simulink model "Pacemaker_model_assgn2"  (R2019a)
settings: Solver=FixedStepAuto  StartTime=0.0  StopTime=inf  FixedStep=1e-3  RelTol=1e-3  EnableMultiTasking=on
undefined symbols (not defined in the file): D0, D1, D10, D11, D12, D13, D2, D3, D4, D5, D6, D7, D8, D9, PTA0, PTA1, PTA2, PTB23, PTB9, PTC16, PTC17, PTC2, PTC3, PTC4, PTD0, PTD1, PTD2, PTD3
libraries: frdmk64flib x21, etargetslib x15, dspstat3 x1
settings Model: ExtModeTrigDuration=5  Creator=dr_pa  LastModifiedBy=dr_pa
settings SolverCC: ConcurrentTasks=on
settings OptimizationCC: EnhancedBackFolding=on  PassReuseOutputArgsAs=Individual arguments  MaxStackSize=64  OptimizeBlockOrder=speed  DifferentSizesBufferReuse=on  OptimizationCustomize=off
settings DebuggingCC: ParameterTunabilityLossMsg=error
settings HardwareCC: ProdBitPerPointer=32  ProdBitPerSizeT=32  ProdBitPerPtrDiffT=32  ProdLargestAtomicInteger=Long  ProdLargestAtomicFloat=Double  ProdWordSize=32  ProdHWDeviceType=ARM Compatible->ARM Cortex
settings SFSimCC: MATLABDynamicMemAlloc=off
settings RTWCC: SystemTargetFile=ert.tlc  HardwareBoard=NXP FRDM-K64F  TLCOptions="-aInlineSetEventsForThisBaseRateFcn=TLC_FALSE -aSuppressMultiTaskScheduler=TLC_FALSE  -aRateBasedStepFcn=0"  TemplateMakefile=ert_default_tmf  GenerateReport=on  Toolchain=GNU Tools for ARM Embedded Processors  BuildConfiguration=Faster Runs  IncludeHyperlinkInReport=on  LaunchReport=on  GenerateTraceInfo=on  GenerateTraceReport=on  GenerateTraceReportSl=on  GenerateTraceReportSf=on  GenerateTraceReportEml=on
settings CodeAppCC: ForceParamTrailComments=on  IgnoreCustomStorageClasses=off  OperatorAnnotations=on  SimulinkDataObjDesc=on  SFDataObjDesc=on  InsertBlockDesc=on

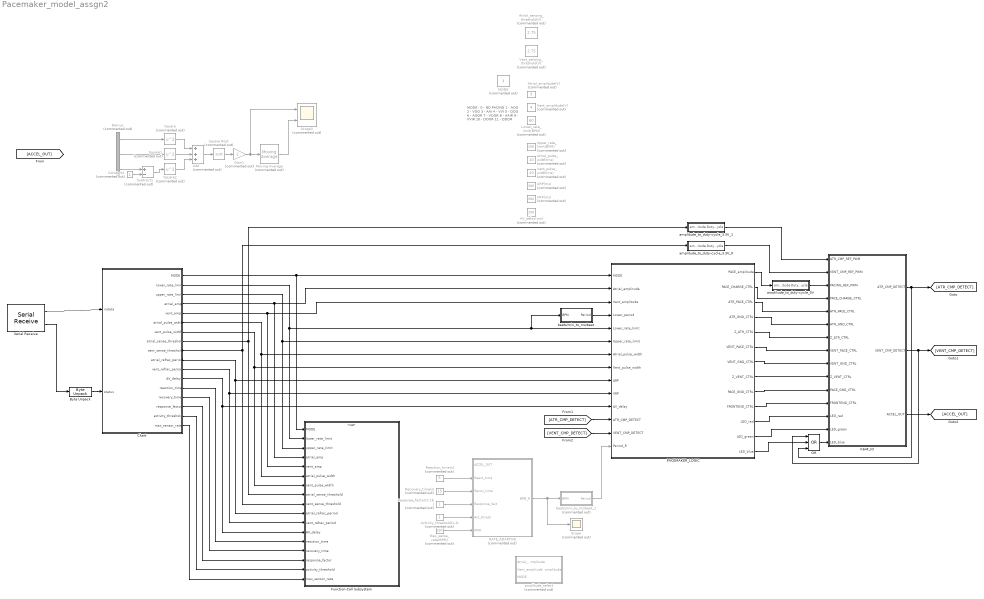
== system Pacemaker_model_assgn2 ==
  note: MODE :
      | 0 - NO PACING
      | 1 - AOO
      | 2 - VOO
      | 3 - AAI
      | 4 - VVI
      | 5 - DOO
      | 6 - AOOR
      | 7 - VOOR
      | 8 - AAIR
      | 9 - VVIR
      | 10 - DOOR
      | 11 - DDDR
  ARP(ms) : Constant  Commented=on  Value=300  OutDataTypeStr=uint16
  AV_delay(ms) : Constant  Commented=on  Value=150  OutDataTypeStr=uint16
  Activity_threshold(1-4) : Constant  Commented=on  OutDataTypeStr=uint8
  Add : Sum  Commented=on  Inputs=+++  AccumDataTypeStr=double  OutDataTypeStr=double
  Atrial_amplitude(V) : Constant  Commented=on  Value=3  OutDataTypeStr=double
  Atrial_pulse_width(ms) : Constant  Commented=on  Value=10  OutDataTypeStr=uint16
  Atrial_sensing_threshold(V) : Constant  Commented=on  Value=2.75  OutDataTypeStr=double
  Byte Unpack : etargetslib/Byte Unpack  dimensions={[1]}  datatypes={'uint8'}  byteAlign=1
      settings: SourceProductName=MATLAB Coder
  Chart : Stateflow chart  BlockKeywords=__PRM__SERIALIZED__DATA__:Stateflow Chart,Stateflow Diagram  TreatAsAtomicUnit=on
  Constant1 : Constant  Commented=on  OutDataTypeStr=double
  Demux : Demux  Commented=on  Outputs=3
  Function-Call Subsystem : Subsystem  TreatAsAtomicUnit=on
  Gain1 : Gain  Commented=on  Gain=2  ParamDataTypeStr=double  OutDataTypeStr=double
  K64F_IO : Subsystem
  Lower_rate_limit(BPM) : Constant  Commented=on  Value=60  OutDataTypeStr=uint16
  MODE : Constant  Commented=on  Value=3  OutDataTypeStr=uint8
  Max_sense_rate(BPM) : Constant  Commented=on  Value=120  OutDataTypeStr=uint16
  Moving Average : dspstat3/Moving Average  Commented=on  Method=Sliding window  ForgettingFactorPort=off  SpecifyWindowLength=on  WindowLength=25  ForgettingFactor=0.9  SimulateUsing=Code generation
  OR : Logic  Operator=OR  Inputs=3  IconShape=distinctive  AllPortsSameDT=off  OutDataTypeStr=boolean
  PACEMAKER_LOGIC : Stateflow chart  BlockKeywords=__PRM__SERIALIZED__DATA__:Stateflow Chart,Stateflow Diagram  TreatAsAtomicUnit=on
  RATE_ADAPTIVE : Subsystem  Commented=on
  Reaction_time(s) : Constant  Commented=on  Value=5  OutDataTypeStr=uint16
  Recovery_time(s) : Constant  Commented=on  Value=15  OutDataTypeStr=uint16
  Response_factor(1-16) : Constant  Commented=on  OutDataTypeStr=uint8
  Scope : Scope  Commented=on
  Scope3 : Scope  Commented=on  NumInputPorts=2
  Serial Receive : frdmk64flib/Serial Receive  SCIModule=0  Baudrate=uint32(9600)  Parity=None  StopBits=1  HardwareFlowControl=None  ByteOrder=LittleEndian  DataType=uint8  DataLength=55  BlockingMode=off  OutputStatus=on  SampleTime=-1
      settings: SourceProductName=Simulink Coder Support Package for NXP FRDM-K64F Board
  Square : Math  Commented=on  Operator=square  OutDataTypeStr=double  SaturateOnIntegerOverflow=on
  Square Root : Sqrt  Commented=on  OutDataTypeStr=double  IntermediateResultsDataTypeStr=double  SaturateOnIntegerOverflow=on
  Square1 : Math  Commented=on  Operator=square  OutDataTypeStr=double  SaturateOnIntegerOverflow=on
  Square2 : Math  Commented=on  Operator=square  OutDataTypeStr=double  SaturateOnIntegerOverflow=on
  Subtract1 : Sum  Commented=on  Inputs=+-  AccumDataTypeStr=double
  Upper_rate_limit(BPM) : Constant  Commented=on  Value=150  OutDataTypeStr=uint16
  VRP(ms) : Constant  Commented=on  Value=300  OutDataTypeStr=uint16
  Vent_amplitude(V) : Constant  Commented=on  Value=4  OutDataTypeStr=double
  Vent_pulse_width(ms) : Constant  Commented=on  Value=10  OutDataTypeStr=uint16
  Vent_sensing_threshold(V) : Constant  Commented=on  Value=2.75  OutDataTypeStr=double
  amplitude_select : Subsystem  Commented=on
  amplitude_to_duty-cycle_3.3V_0 : Subsystem
  amplitude_to_duty-cycle_3.3V_1 : Subsystem
  amplitude_to_duty-cycle_5V : Subsystem
  beats/min_to_ms/beat : Subsystem
  beats/min_to_ms/beat_1 : Subsystem  Commented=on
  wires:
  PACEMAKER_LOGIC/9(PACE_GND_CTRL) -> K64F_IO/11(PACE_GND_CTRL)
  PACEMAKER_LOGIC/8(Z_VENT_CTRL) -> K64F_IO/10(Z_VENT_CTRL)
  PACEMAKER_LOGIC/7(VENT_GND_CTRL) -> K64F_IO/9(VENT_GND_CTRL)
  PACEMAKER_LOGIC/6(VENT_PACE_CTRL) -> K64F_IO/8(VENT_PACE_CTRL)
  PACEMAKER_LOGIC/5(Z_ATR_CTRL) -> K64F_IO/7(Z_ATR_CTRL)
  PACEMAKER_LOGIC/4(ATR_GND_CTRL) -> K64F_IO/6(ATR_GND_CTRL)
  PACEMAKER_LOGIC/3(ATR_PACE_CTRL) -> K64F_IO/5(ATR_PACE_CTRL)
  PACEMAKER_LOGIC/2(PACE_CHARGE_CTRL) -> K64F_IO/4(PACE_CHARGE_CTRL)
  amplitude_to_duty-cycle_5V/1(Duty Cycle) -> K64F_IO/3(PACING_REF_PWM)
  beats/min_to_ms/beat/1(Period) -> PACEMAKER_LOGIC/4(Lower_period)
  amplitude_to_duty-cycle_3.3V_0/1(Duty Cycle) -> K64F_IO/2(VENT_CMP_REF_PWM)
  amplitude_to_duty-cycle_3.3V_1/1(Duty Cycle) -> K64F_IO/1(ATR_CMP_REF_PWM)
  PACEMAKER_LOGIC/10(FRONTEND_CTRL) -> K64F_IO/12(FRONTEND_CTRL)
  PACEMAKER_LOGIC/12(LED_green) -> K64F_IO/14(LED_green)
  PACEMAKER_LOGIC/11(LED_red) -> K64F_IO/13(LED_red)
  PACEMAKER_LOGIC/13(LED_blue) -> OR/2
  PACEMAKER_LOGIC/1(PACE_amplitude) -> amplitude_to_duty-cycle_5V/1(amplitude)
  K64F_IO/1(ATR_CMP_DETECT) -> [ATR_CMP_DETECT], OR/3
  [ATR_CMP_DETECT] -> PACEMAKER_LOGIC/12(ATR_CMP_DETECT)
  K64F_IO/2(VENT_CMP_DETECT) -> [VENT_CMP_DETECT], OR/1
  [VENT_CMP_DETECT] -> PACEMAKER_LOGIC/13(VENT_CMP_DETECT)
  K64F_IO/3(ACCEL_OUT) -> [ACCEL_OUT]
  RATE_ADAPTIVE/1(BPM_R) -> Scope/1, beats/min_to_ms/beat_1/1(BPM)
  beats/min_to_ms/beat_1/1(Period) -> PACEMAKER_LOGIC/14(Period_R)
  Reaction_time(s)/1 -> RATE_ADAPTIVE/2(React_time)
  Recovery_time(s)/1 -> RATE_ADAPTIVE/3(Recov_time)
  Response_factor(1-16)/1 -> RATE_ADAPTIVE/4(Response_fact)
  Activity_threshold(1-4)/1 -> RATE_ADAPTIVE/5(Act_thresh)
  Max_sense_rate(BPM)/1 -> RATE_ADAPTIVE/6(MSR)
  OR/1 -> K64F_IO/15(LED_blue)
  Gain1/1 -> Moving Average/1, Scope3/1
  Square Root/1 -> Gain1/1
  Square/1 -> Add/1
  Square2/1 -> Add/3
  Constant1/1 -> Subtract1/2
  Demux/1 -> Square/1
  Square1/1 -> Add/2
  Demux/2 -> Square1/1
  Subtract1/1 -> Square2/1
  Demux/3 -> Subtract1/1
  Moving Average/1 -> Scope3/2
  Add/1 -> Square Root/1
  Chart/11(vent_refrac_period) -> PACEMAKER_LOGIC/10(VRP), Function-Call Subsystem/11(vent_refrac_period)
  Chart/2(lower_rate_limit) -> beats/min_to_ms/beat/1(BPM), PACEMAKER_LOGIC/5(Lower_rate_limit), Function-Call Subsystem/2(lower_rate_limit)
  Serial Receive/1 -> Chart/1(rxdata)
  Chart/9(vent_sense_threshold) -> amplitude_to_duty-cycle_3.3V_0/1(amplitude), Function-Call Subsystem/9(vent_sense_threshold)
  Chart/10(atrial_refrac_period) -> PACEMAKER_LOGIC/9(ARP), Function-Call Subsystem/10(atrial_refrac_period)
  Chart/8(atrial_sense_threshold) -> amplitude_to_duty-cycle_3.3V_1/1(amplitude), Function-Call Subsystem/8(atrial_sense_threshold)
  Chart/7(vent_pulse_width) -> PACEMAKER_LOGIC/8(Vent_pulse_width), Function-Call Subsystem/7(vent_pulse_width)
  Chart/13(reaction_time) -> Function-Call Subsystem/13(reaction_time)
  Chart/15(response_factor) -> Function-Call Subsystem/15(response_factor)
  Chart/4(atrial_amp) -> Function-Call Subsystem/4(atrial_amp), PACEMAKER_LOGIC/2(Atrial_amplitude)
  Chart/12(AV_delay) -> PACEMAKER_LOGIC/11(AV_delay), Function-Call Subsystem/12(AV_delay)
  Chart/1(MODE) -> Function-Call Subsystem/1(MODE), PACEMAKER_LOGIC/1(MODE)
  Chart/6(atrial_pulse_width) -> PACEMAKER_LOGIC/7(Atrial_pulse_width), Function-Call Subsystem/6(atrial_pulse_width)
  Chart/3(upper_rate_limit) -> PACEMAKER_LOGIC/6(Upper_rate_limit), Function-Call Subsystem/3(upper_rate_limit)
  Chart/16(activity_threshold) -> Function-Call Subsystem/16(activity_threshold)
  Chart/5(vent_amp) -> PACEMAKER_LOGIC/3(Vent_amplitude), Function-Call Subsystem/5(vent_amp)
  Chart/17(max_sensor_rate) -> Function-Call Subsystem/17(max_sensor_rate)
  Chart/14(recovery_time) -> Function-Call Subsystem/14(recovery_time)
  Byte Unpack/1 -> Chart/2(status)
  Serial Receive/2 -> Byte Unpack/1

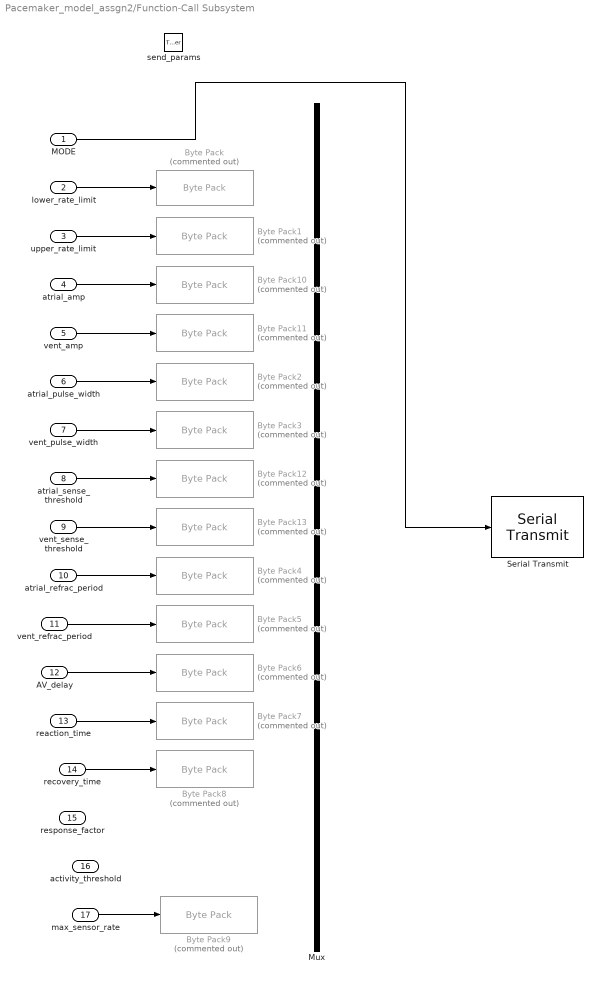
== system Pacemaker_model_assgn2/Function-Call Subsystem ==
  MODE : Inport
  lower_rate_limit : Inport  Port=2
  upper_rate_limit : Inport  Port=3
  atrial_amp : Inport  Port=4
  vent_amp : Inport  Port=5
  atrial_pulse_width : Inport  Port=6
  vent_pulse_width : Inport  Port=7
  atrial_sense_threshold : Inport  Port=8
  vent_sense_threshold : Inport  Port=9
  atrial_refrac_period : Inport  Port=10
  vent_refrac_period : Inport  Port=11
  AV_delay : Inport  Port=12
  reaction_time : Inport  Port=13
  recovery_time : Inport  Port=14
  response_factor : Inport  Port=15
  activity_threshold : Inport  Port=16
  max_sensor_rate : Inport  Port=17
  send_params : TriggerPort  TriggerType=function-call  IsSimulinkFunction=on  FunctionName=send_params  VariantControl=Variant
  Byte Pack{,1..9} (10 alike) : etargetslib/Byte Pack  Commented=on  datatypes={'uint16'}  byteAlign=1
      settings: SourceProductName=MATLAB Coder
  Byte Pack{10..13} (4 alike) : etargetslib/Byte Pack  Commented=on  datatypes={'double'}  byteAlign=1
      settings: SourceProductName=MATLAB Coder
  Mux : Mux  Inputs=17
  Serial Transmit : frdmk64flib/Serial Transmit  SCIModule=0  Baudrate=uint32(9600)  Parity=None  StopBits=1  HardwareFlowControl=None  ByteOrder=LittleEndian  BlockingMode=on  OutputStatus=off
      settings: SourceProductName=Simulink Coder Support Package for NXP FRDM-K64F Board
  wires:
  max_sensor_rate/1 -> Byte Pack9/1
  AV_delay/1 -> Byte Pack6/1
  vent_refrac_period/1 -> Byte Pack5/1
  recovery_time/1 -> Byte Pack8/1
  vent_sense_threshold/1 -> Byte Pack13/1
  atrial_refrac_period/1 -> Byte Pack4/1
  upper_rate_limit/1 -> Byte Pack1/1
  vent_amp/1 -> Byte Pack11/1
  atrial_amp/1 -> Byte Pack10/1
  reaction_time/1 -> Byte Pack7/1
  atrial_pulse_width/1 -> Byte Pack2/1
  atrial_sense_threshold/1 -> Byte Pack12/1
  lower_rate_limit/1 -> Byte Pack/1
  vent_pulse_width/1 -> Byte Pack3/1
  MODE/1 -> Serial Transmit/1

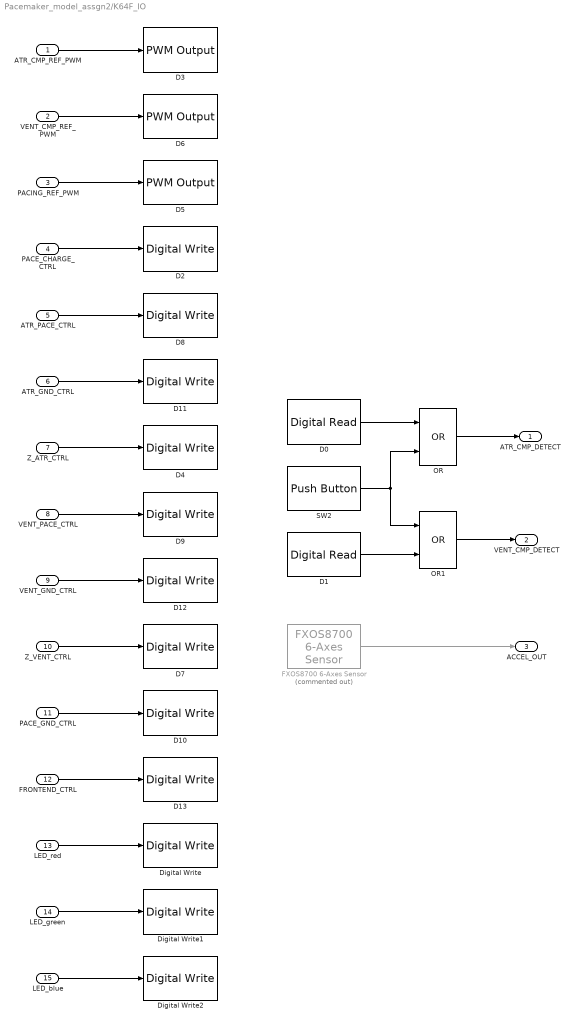
== system Pacemaker_model_assgn2/K64F_IO ==
  ATR_CMP_REF_PWM : Inport  OutDataTypeStr=uint8
  VENT_CMP_REF_PWM : Inport  Port=2  OutDataTypeStr=uint8
  PACING_REF_PWM : Inport  Port=3  OutDataTypeStr=uint8
  PACE_CHARGE_CTRL : Inport  Port=4  OutDataTypeStr=boolean
  ATR_PACE_CTRL : Inport  Port=5  OutDataTypeStr=boolean
  ATR_GND_CTRL : Inport  Port=6  OutDataTypeStr=boolean
  Z_ATR_CTRL : Inport  Port=7  OutDataTypeStr=boolean
  VENT_PACE_CTRL : Inport  Port=8  OutDataTypeStr=boolean
  VENT_GND_CTRL : Inport  Port=9  OutDataTypeStr=boolean
  Z_VENT_CTRL : Inport  Port=10  OutDataTypeStr=boolean
  PACE_GND_CTRL : Inport  Port=11  OutDataTypeStr=boolean
  FRONTEND_CTRL : Inport  Port=12  OutDataTypeStr=boolean
  LED_red : Inport  Port=13  OutDataTypeStr=boolean
  LED_green : Inport  Port=14  OutDataTypeStr=boolean
  LED_blue : Inport  Port=15  OutDataTypeStr=boolean
  D0 : frdmk64flib/Digital Read  Whichpin=PTC16 (D0)  SampleTime=-1
      settings: SourceProductName=Simulink Coder Support Package for NXP FRDM-K64F Board
  D1 : frdmk64flib/Digital Read  Whichpin=PTC17 (D1)  SampleTime=-1
      settings: SourceProductName=Simulink Coder Support Package for NXP FRDM-K64F Board
  D10 : frdmk64flib/Digital Write  Whichpin=PTD0 (D10)
      settings: SourceProductName=Simulink Coder Support Package for NXP FRDM-K64F Board
  D11 : frdmk64flib/Digital Write  Whichpin=PTD2 (D11)
      settings: SourceProductName=Simulink Coder Support Package for NXP FRDM-K64F Board
  D12 : frdmk64flib/Digital Write  Whichpin=PTD3 (D12)
      settings: SourceProductName=Simulink Coder Support Package for NXP FRDM-K64F Board
  D13 : frdmk64flib/Digital Write  Whichpin=PTD1 (D13)
      settings: SourceProductName=Simulink Coder Support Package for NXP FRDM-K64F Board
  D2 : frdmk64flib/Digital Write  Whichpin=PTB9 (D2)
      settings: SourceProductName=Simulink Coder Support Package for NXP FRDM-K64F Board
  D3 : frdmk64flib/PWM Output  Whichpin=PTA1 (D3)  InitialFrequency=2000  InitialDutyCycle=0
      settings: SourceProductName=Simulink Coder Support Package for NXP FRDM-K64F Board
  D4 : frdmk64flib/Digital Write  Whichpin=PTB23 (D4)
      settings: SourceProductName=Simulink Coder Support Package for NXP FRDM-K64F Board
  D5 : frdmk64flib/PWM Output  Whichpin=PTA2 (D5)  InitialFrequency=2000  InitialDutyCycle=0
      settings: SourceProductName=Simulink Coder Support Package for NXP FRDM-K64F Board
  D6 : frdmk64flib/PWM Output  Whichpin=PTC2 (D6)  InitialFrequency=2000  InitialDutyCycle=0
      settings: SourceProductName=Simulink Coder Support Package for NXP FRDM-K64F Board
  D7 : frdmk64flib/Digital Write  Whichpin=PTC3 (D7)
      settings: SourceProductName=Simulink Coder Support Package for NXP FRDM-K64F Board
  D8 : frdmk64flib/Digital Write  Whichpin=PTA0 (D8)
      settings: SourceProductName=Simulink Coder Support Package for NXP FRDM-K64F Board
  D9 : frdmk64flib/Digital Write  Whichpin=PTC4 (D9)
      settings: SourceProductName=Simulink Coder Support Package for NXP FRDM-K64F Board
  Digital Write : frdmk64flib/Digital Write  Whichpin=RED_LED
      settings: SourceProductName=Simulink Coder Support Package for NXP FRDM-K64F Board
  Digital Write1 : frdmk64flib/Digital Write  Whichpin=GREEN_LED
      settings: SourceProductName=Simulink Coder Support Package for NXP FRDM-K64F Board
  Digital Write2 : frdmk64flib/Digital Write  Whichpin=BLUE_LED
      settings: SourceProductName=Simulink Coder Support Package for NXP FRDM-K64F Board
  FXOS8700 6-Axes Sensor : frdmk64flib/FXOS8700 6-Axes Sensor  Commented=on  Activesensor=Accelerometer only  ODR=200Hz  HybridODR=100Hz  Accelfullrange=-4g to +4g  SampleTime=10e-3
      settings: SourceProductName=Simulink Coder Support Package for NXP FRDM-K64F Board
  OR : Logic  Operator=OR  IconShape=distinctive  AllPortsSameDT=off  OutDataTypeStr=boolean
  OR1 : Logic  Operator=OR  IconShape=distinctive  AllPortsSameDT=off  OutDataTypeStr=boolean
  SW2 : frdmk64flib/Push Button  Whichswitch=SW2  SampleTime1=-1
      settings: SourceProductName=Simulink Coder Support Package for NXP FRDM-K64F Board
  ATR_CMP_DETECT : Outport  OutDataTypeStr=boolean
  VENT_CMP_DETECT : Outport  Port=2  OutDataTypeStr=boolean
  ACCEL_OUT : Outport  Port=3  OutDataTypeStr=double
  wires:
  PACING_REF_PWM/1 -> D5/1
  PACE_CHARGE_CTRL/1 -> D2/1
  VENT_PACE_CTRL/1 -> D9/1
  VENT_GND_CTRL/1 -> D12/1
  ATR_PACE_CTRL/1 -> D8/1
  ATR_GND_CTRL/1 -> D11/1
  PACE_GND_CTRL/1 -> D10/1
  Z_ATR_CTRL/1 -> D4/1
  Z_VENT_CTRL/1 -> D7/1
  FRONTEND_CTRL/1 -> D13/1
  ATR_CMP_REF_PWM/1 -> D3/1
  VENT_CMP_REF_PWM/1 -> D6/1
  LED_red/1 -> Digital Write/1
  LED_green/1 -> Digital Write1/1
  D0/1 -> OR/1
  D1/1 -> OR1/2
  SW2/1 -> OR/2, OR1/1
  OR/1 -> ATR_CMP_DETECT/1
  OR1/1 -> VENT_CMP_DETECT/1
  LED_blue/1 -> Digital Write2/1
  FXOS8700 6-Axes Sensor/1 -> ACCEL_OUT/1

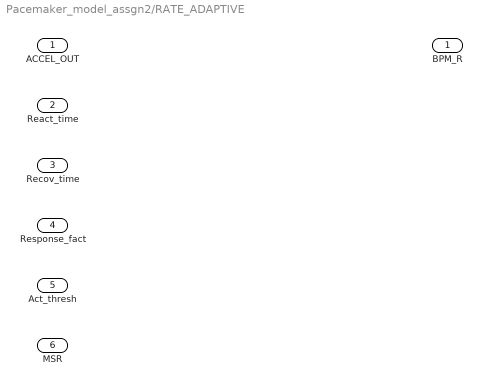
== system Pacemaker_model_assgn2/RATE_ADAPTIVE ==
  ACCEL_OUT : Inport  OutDataTypeStr=double
  React_time : Inport  Port=2  OutDataTypeStr=uint16
  Recov_time : Inport  Port=3  OutDataTypeStr=uint16
  Response_fact : Inport  Port=4  OutDataTypeStr=uint8
  Act_thresh : Inport  Port=5  OutDataTypeStr=uint8
  MSR : Inport  Port=6  OutDataTypeStr=uint16
  BPM_R : Outport

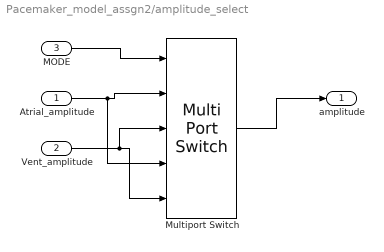
== system Pacemaker_model_assgn2/amplitude_select ==
  Atrial_amplitude : Inport  OutDataTypeStr=double
  Vent_amplitude : Inport  Port=2  OutDataTypeStr=double
  MODE : Inport  Port=3  OutDataTypeStr=uint8
  Multiport Switch : MultiPortSwitch  DataPortOrder=Zero-based contiguous  Inputs=4  zeroidx=on
  amplitude : Outport  OutDataTypeStr=double
  wires:
  Multiport Switch/1 -> amplitude/1
  MODE/1 -> Multiport Switch/1
  Atrial_amplitude/1 -> Multiport Switch/4, Multiport Switch/2
  Vent_amplitude/1 -> Multiport Switch/5, Multiport Switch/3

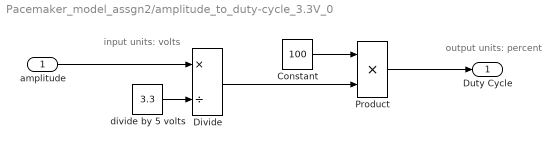
== system Pacemaker_model_assgn2/amplitude_to_duty-cycle_3.3V_0 ==
  note: input units: volts
  note: output units: percent
  amplitude : Inport  OutDataTypeStr=double
  Constant : Constant  Value=100  OutDataTypeStr=double
  Divide : Product  Inputs=*/  OutDataTypeStr=double
  Product : Product  OutDataTypeStr=uint8  RndMeth=Round
  divide by 5 volts : Constant  Value=3.3  OutDataTypeStr=double
  Duty Cycle : Outport  OutDataTypeStr=uint8
  wires:
  amplitude/1 -> Divide/1
  Product/1 -> Duty Cycle/1
  Constant/1 -> Product/1
  Divide/1 -> Product/2
  divide by 5 volts/1 -> Divide/2

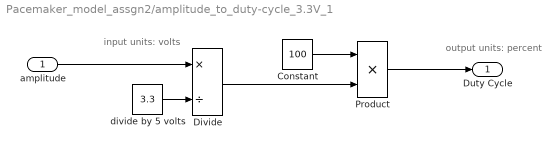
== system Pacemaker_model_assgn2/amplitude_to_duty-cycle_3.3V_1 ==
  note: output units: percent
  note: input units: volts
  amplitude : Inport  OutDataTypeStr=double
  Constant : Constant  Value=100  OutDataTypeStr=double
  Divide : Product  Inputs=*/  OutDataTypeStr=double
  Product : Product  OutDataTypeStr=uint8  RndMeth=Round
  divide by 5 volts : Constant  Value=3.3  OutDataTypeStr=double
  Duty Cycle : Outport  OutDataTypeStr=uint8
  wires:
  divide by 5 volts/1 -> Divide/2
  Divide/1 -> Product/2
  Constant/1 -> Product/1
  Product/1 -> Duty Cycle/1
  amplitude/1 -> Divide/1

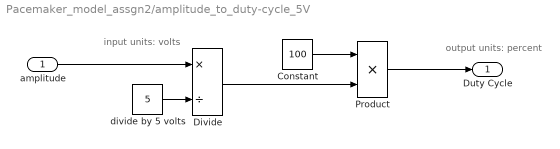
== system Pacemaker_model_assgn2/amplitude_to_duty-cycle_5V ==
  note: output units: percent
  note: input units: volts
  amplitude : Inport  OutDataTypeStr=double
  Constant : Constant  Value=100  OutDataTypeStr=double
  Divide : Product  Inputs=*/  OutDataTypeStr=double
  Product : Product  OutDataTypeStr=uint8  RndMeth=Round
  divide by 5 volts : Constant  Value=5  OutDataTypeStr=double
  Duty Cycle : Outport  OutDataTypeStr=uint8
  wires:
  divide by 5 volts/1 -> Divide/2
  Divide/1 -> Product/2
  Constant/1 -> Product/1
  Product/1 -> Duty Cycle/1
  amplitude/1 -> Divide/1

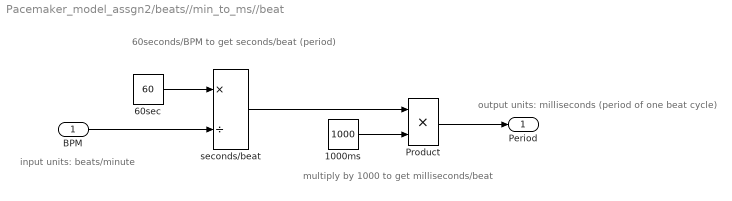
== system Pacemaker_model_assgn2/beats//min_to_ms//beat ==
  note: input units: beats/minute
  note: output units: milliseconds (period of one beat cycle)
  note: 60seconds/BPM to get seconds/beat (period)
  note: multiply by 1000 to get milliseconds/beat
  BPM : Inport  OutDataTypeStr=uint16
  1000ms : Constant  Value=1000  OutDataTypeStr=double
  60sec : Constant  Value=60  OutDataTypeStr=double
  Product : Product  OutDataTypeStr=uint16  RndMeth=Round
  seconds/beat : Product  Inputs=*/  OutDataTypeStr=double
  Period : Outport  OutDataTypeStr=uint16
  wires:
  1000ms/1 -> Product/2
  Product/1 -> Period/1
  seconds/beat/1 -> Product/1
  60sec/1 -> seconds/beat/1
  BPM/1 -> seconds/beat/2

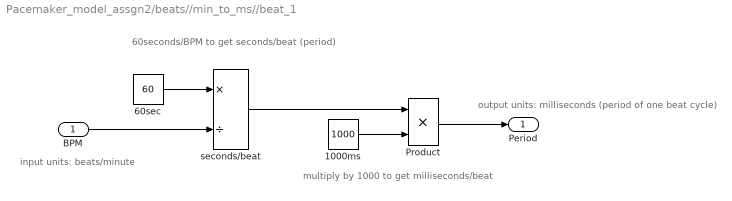
== system Pacemaker_model_assgn2/beats//min_to_ms//beat_1 ==
  note: input units: beats/minute
  note: output units: milliseconds (period of one beat cycle)
  note: 60seconds/BPM to get seconds/beat (period)
  note: multiply by 1000 to get milliseconds/beat
  BPM : Inport  OutDataTypeStr=uint16
  1000ms : Constant  Value=1000  OutDataTypeStr=double
  60sec : Constant  Value=60  OutDataTypeStr=double
  Product : Product  OutDataTypeStr=uint16  RndMeth=Round
  seconds/beat : Product  Inputs=*/  OutDataTypeStr=double
  Period : Outport  OutDataTypeStr=uint16
  wires:
  1000ms/1 -> Product/2
  Product/1 -> Period/1
  seconds/beat/1 -> Product/1
  60sec/1 -> seconds/beat/1
  BPM/1 -> seconds/beat/2

== stateflow chart Pacemaker_model_assgn2/Chart ==
  state SET_PARAMS
    %we assume this is the order that the data is sent in
    entry:
    %MODE = rxdata(1);
    %lower_rate_limit = typecast(rxdata(2:3), 'uint16');
    %upper_rate_limit = typecast(rxdata(4:5), 'uint16');
    %atrial_amp = typecast(rxdata(6:13), 'double');
    %vent_amp = typecast(rxdata(14:21), 'double');
    %atrial_pulse_width = typecast(rxdata(22:23), 'uint16');
    %vent_pulse_width = typecast(rxdata(24:25), 'uint16')
    %atrial_sense_threshold = typecast(rxdata(26:33), 'double')
    %vent_sense_threshold = typecast(rxdata(34:41), 'double')
    %atrial_refrac_period = typecast(rxdata(42:43), 'uint16')
    %vent_refrac_period = typecast(rxdata(44:45), 'uint16')
    %AV_delay = typecast(rxdata(46:47), 'uint16')
    %reaction_time = typecast(rxdata(48:49), 'uint16')
    %recovery_time = typecast(rxdata(50:51), 'uint16')
    %response_factor = rxdata(52)
    %activity_threshold = rxdata(53)
    %max_sensor_rate = typecast(rxdata(54:55), 'uint16')
    send_params();
  note: transmitting DCM to board is if 0xFF
      | receiving board to DCM is 0x05
  state INITIAL
    entry:
    MODE = 1;
    lower_rate_limit = 60;
    upper_rate_limit = 120;
    atrial_amp = 3.3;
    vent_amp = 3.3;
    atrial_pulse_width = 10;
    vent_pulse_width = 10;
    atrial_sense_threshold = 2.75;
    vent_sense_threshold = 2.75;
    atrial_refrac_period = 300;
    vent_refrac_period = 300;
    AV_delay = 100;
    reaction_time = 0; %unknown
    recovery_time = 0; %unknown
    response_factor = 0; %unknown
    activity_threshold = 0; %unknown
    max_sensor_rate = 0; %unknown
  state STANDBY
    %Waiting for COM
  note: status == 0 indicates successful read
  state SEND_PARAMS
    entry:
    send_params();
  (default) -> INITIAL
  SET_PARAMS -> STANDBY
  STANDBY -> SET_PARAMS [order 2] : [status == 0]
  INITIAL -> STANDBY
  STANDBY -> SEND_PARAMS [order 1] : [rxdata(56) == hex2dec('05') && status == 0]
  SEND_PARAMS -> STANDBY
  data: rxdata input uint8; status input uint8; MODE output uint8; lower_rate_limit output uint16; upper_rate_limit output uint16; atrial_amp output double; vent_amp output double; atrial_pulse_width output uint16; vent_pulse_width output uint16; atrial_sense_threshold output double; vent_sense_threshold output double; atrial_refrac_period output uint16; vent_refrac_period output uint16; AV_delay output uint16; reaction_time output uint16; recovery_time output uint16; response_factor output uint8; activity_threshold output uint8; max_sensor_rate output uint16

== stateflow chart Pacemaker_model_assgn2/PACEMAKER_LOGIC ==
  state AOO [group]
    state AOO_PACE_ATRIUM
      entry:
      LED_green = true;
      PACE_CHARGE_CTRL = false;
      PACE_GND_CTRL = true;
      VENT_PACE_CTRL = false;
      VENT_GND_CTRL = false;
      Z_VENT_CTRL = false;
      Z_ATR_CTRL = false;
      ATR_GND_CTRL = false;
      ATR_PACE_CTRL = true;
    state AOO_DischargeC21_ChargeC22
      entry:
      LED_red = false;
      LED_green = false;
      PACE_amplitude = Atrial_amplitude;
      PACE_GND_CTRL = true;
      ATR_PACE_CTRL = false;
      Z_ATR_CTRL = false;
      Z_VENT_CTRL = false;
      VENT_PACE_CTRL = false;
      VENT_GND_CTRL = false;
      ATR_GND_CTRL = true;
      PACE_CHARGE_CTRL = true;
    AOO_DischargeC21_ChargeC22 -> AOO_PACE_ATRIUM [order 1] : after((Lower_period-Atrial_pulse_width), msec)
    AOO_PACE_ATRIUM -> AOO_DischargeC21_ChargeC22 : after(Atrial_pulse_width, msec)
  state VOO [group]
    state VOO_PACE_VENT
      entry:
      LED_green = true;
      PACE_CHARGE_CTRL = false;
      PACE_GND_CTRL = true;
      ATR_PACE_CTRL = false;
      ATR_GND_CTRL = false;
      Z_ATR_CTRL = false;
      Z_VENT_CTRL = false;
      VENT_GND_CTRL = false;
      VENT_PACE_CTRL = true;
    state VOO_DischargeC21_ChargeC22
      entry:
      LED_red = false;
      LED_green = false;
      PACE_amplitude = Vent_amplitude;
      PACE_GND_CTRL = true;
      VENT_PACE_CTRL = false;
      Z_VENT_CTRL = false;
      Z_ATR_CTRL = false;
      ATR_PACE_CTRL = false;
      ATR_GND_CTRL = false;
      VENT_GND_CTRL = true;
      PACE_CHARGE_CTRL = true;
    VOO_DischargeC21_ChargeC22 -> VOO_PACE_VENT [order 1] : after((Lower_period-Vent_pulse_width), msec)
    VOO_PACE_VENT -> VOO_DischargeC21_ChargeC22 : after(Vent_pulse_width, msec)
  state AAI [group] [commented out]
    state ARP [commented out]
      entry:
      LED_green = false;
      PACE_GND_CTRL = true;
      ATR_PACE_CTRL = false;
      Z_ATR_CTRL = false;
      Z_VENT_CTRL = false;
      VENT_PACE_CTRL = false;
      VENT_GND_CTRL = false;
      ATR_GND_CTRL = true;
      PACE_CHARGE_CTRL = true;
    state AAI_PACE_ATRIUM [commented out]
      entry:
      FRONTEND_CTRL = false;
      LED_green = true;
      PACE_CHARGE_CTRL = false;
      PACE_GND_CTRL = true;
      VENT_PACE_CTRL = false;
      VENT_GND_CTRL = false;
      Z_VENT_CTRL = false;
      Z_ATR_CTRL = false;
      ATR_GND_CTRL = false;
      ATR_PACE_CTRL = true;
    state AAI_DischargeC21_ChargeC22 [commented out]
      entry:
      FRONTEND_CTRL = true;
      LED_blue = false;
      LED_red = false;
      LED_green = false;
      PACE_GND_CTRL = true;
      ATR_PACE_CTRL = false;
      Z_ATR_CTRL = false;
      Z_VENT_CTRL = false;
      VENT_PACE_CTRL = false;
      VENT_GND_CTRL = false;
      ATR_GND_CTRL = true;
      PACE_CHARGE_CTRL = true;
    AAI.AAI_PACE_ATRIUM -> AAI.ARP [commented out] : after(Atrial_pulse_width, msec)
    AAI.AAI_DischargeC21_ChargeC22 -> AAI.ARP [commented out] : [ATR_CMP_DETECT==true]
    AAI.ARP -> AAI.AAI_DischargeC21_ChargeC22 [commented out] : after(ARP, msec)
    AAI.AAI_DischargeC21_ChargeC22 -> AAI.AAI_PACE_ATRIUM [commented out] : after((Lower_period-Atrial_pulse_width-ARP), msec)
  state HOLD
    entry:
    PACE_CHARGE_CTRL = false;
    PACE_GND_CTRL = false;
    ATR_GND_CTRL = false;
    VENT_GND_CTRL = false;
    ATR_PACE_CTRL = false;
    VENT_PACE_CTRL = false;
    FRONTEND_CTRL = true;
    LED_red = true;
    LED_green = false;
    LED_blue = false;
    APW_delay = 0;
    VPW_delay = 0;
  state AAI [group]
    state ARP
      entry:
      PACE_GND_CTRL = true;
      ATR_PACE_CTRL = false;
      Z_ATR_CTRL = false;
      Z_VENT_CTRL = false;
      VENT_PACE_CTRL = false;
      VENT_GND_CTRL = false;
      ATR_GND_CTRL = true;
      PACE_CHARGE_CTRL = true;
      FRONTEND_CTRL = true;
      LED_green = false;
    state AAI_PACE_ATRIUM
      entry:
      PACE_CHARGE_CTRL = false;
      PACE_GND_CTRL = true;
      VENT_PACE_CTRL = false;
      VENT_GND_CTRL = false;
      Z_VENT_CTRL = false;
      Z_ATR_CTRL = false;
      ATR_GND_CTRL = false;
      FRONTEND_CTRL = false;
      ATR_PACE_CTRL = true;
      APW_delay = Atrial_pulse_width;
      LED_green = true;
    state AAI_DischargeC21_ChargeC22
      entry:
      PACE_amplitude = Atrial_amplitude;
      PACE_GND_CTRL = true;
      ATR_PACE_CTRL = false;
      Z_ATR_CTRL = false;
      Z_VENT_CTRL = false;
      VENT_PACE_CTRL = false;
      VENT_GND_CTRL = false;
      ATR_GND_CTRL = true;
      PACE_CHARGE_CTRL = true;
      LED_blue = false;
      LED_red = false;
      LED_green = false;
    AAI.AAI_PACE_ATRIUM -> AAI.ARP : after(Atrial_pulse_width, msec)
    AAI.AAI_DischargeC21_ChargeC22 -> AAI.ARP [order 1] : [ATR_CMP_DETECT==true]
        | {APW_delay = 0;}
    AAI.ARP -> AAI.AAI_DischargeC21_ChargeC22 : after(ARP, msec)
    AAI.AAI_DischargeC21_ChargeC22 -> AAI.AAI_PACE_ATRIUM [order 2] : after((Lower_period-ARP-APW_delay), msec)
  state VVI [group] [commented out]
    state VRP [commented out]
      entry:
      LED_green = false;
      PACE_GND_CTRL = true;
      VENT_PACE_CTRL = false;
      Z_VENT_CTRL = false;
      Z_ATR_CTRL = false;
      ATR_PACE_CTRL = false;
      ATR_GND_CTRL = false;
      VENT_GND_CTRL = true;
      PACE_CHARGE_CTRL = true;
    state VVI_PACE_VENT [commented out]
      entry:
      FRONTEND_CTRL = false;
      LED_green = true;
      PACE_CHARGE_CTRL = false;
      PACE_GND_CTRL = true;
      ATR_PACE_CTRL = false;
      ATR_GND_CTRL = false;
      Z_ATR_CTRL = false;
      Z_VENT_CTRL = false;
      VENT_GND_CTRL = false;
      VENT_PACE_CTRL = true;
    state VVI_DischargeC21_ChargeC22 [commented out]
      entry:
      FRONTEND_CTRL = true;
      LED_blue = false;
      LED_red = false;
      LED_green = false;
      PACE_GND_CTRL = true;
      VENT_PACE_CTRL = false;
      Z_VENT_CTRL = false;
      Z_ATR_CTRL = false;
      ATR_PACE_CTRL = false;
      ATR_GND_CTRL = false;
      VENT_GND_CTRL = true;
      PACE_CHARGE_CTRL = true;
    VVI.VVI_DischargeC21_ChargeC22 -> VVI.VRP [commented out] : [VENT_CMP_DETECT==true]
    VVI.VVI_PACE_VENT -> VVI.VRP [commented out] : after(Vent_pulse_width, msec)
    VVI.VRP -> VVI.VVI_DischargeC21_ChargeC22 [commented out] : after(VRP, msec)
    VVI.VVI_DischargeC21_ChargeC22 -> VVI.VVI_PACE_VENT [commented out] : after(Lower_period-Vent_pulse_width-ARP, msec)
  state VVI [group]
    state VRP
      entry:
      PACE_GND_CTRL = true;
      VENT_PACE_CTRL = false;
      Z_VENT_CTRL = false;
      Z_ATR_CTRL = false;
      ATR_PACE_CTRL = false;
      ATR_GND_CTRL = false;
      VENT_GND_CTRL = true;
      PACE_CHARGE_CTRL = true;
      FRONTEND_CTRL = true;
      LED_green = false;
    state VVI_PACE_VENT
      entry:
      LED_green = true;
      PACE_CHARGE_CTRL = false;
      PACE_GND_CTRL = true;
      ATR_PACE_CTRL = false;
      ATR_GND_CTRL = false;
      Z_ATR_CTRL = false;
      Z_VENT_CTRL = false;
      VENT_GND_CTRL = false;
      FRONTEND_CTRL = false;
      VENT_PACE_CTRL = true;
      VPW_delay = Vent_pulse_width;
    state VVI_DischargeC21_ChargeC22
      entry:
      PACE_amplitude = Vent_amplitude;
      PACE_GND_CTRL = true;
      VENT_PACE_CTRL = false;
      Z_VENT_CTRL = false;
      Z_ATR_CTRL = false;
      ATR_PACE_CTRL = false;
      ATR_GND_CTRL = false;
      VENT_GND_CTRL = true;
      PACE_CHARGE_CTRL = true;
      LED_blue = false;
      LED_red = false;
      LED_green = false;
    VVI.VVI_DischargeC21_ChargeC22 -> VVI.VRP [order 1] : [VENT_CMP_DETECT==true]
        | {VPW_delay = 0;}
    VVI.VVI_PACE_VENT -> VVI.VRP : after(Vent_pulse_width, msec)
    VVI.VRP -> VVI.VVI_DischargeC21_ChargeC22 : after(VRP, msec)
    VVI.VVI_DischargeC21_ChargeC22 -> VVI.VVI_PACE_VENT [order 2] : after(Lower_period-Vent_pulse_width-VPW_delay, msec)
  state DOO [group]
    state VOO_DischargeC21A_ChargeC22V
      entry:
      LED_red = false;
      LED_green = false;
      PACE_amplitude = Atrial_amplitude;
      PACE_GND_CTRL = true;
      VENT_PACE_CTRL = false;
      Z_VENT_CTRL = false;
      Z_ATR_CTRL = false;
      ATR_PACE_CTRL = false;
      ATR_GND_CTRL = false;
      VENT_GND_CTRL = true;
      PACE_CHARGE_CTRL = true;
    state DOO_PACE_ATRIUM
      entry:
      LED_green = true;
      PACE_CHARGE_CTRL = false;
      PACE_GND_CTRL = true;
      VENT_PACE_CTRL = false;
      VENT_GND_CTRL = false;
      Z_VENT_CTRL = false;
      Z_ATR_CTRL = false;
      ATR_GND_CTRL = false;
      ATR_PACE_CTRL = true;
    state DOO_DischargeC21A_ChargeC22V
      entry:
      LED_red = false;
      LED_green = false;
      PACE_amplitude = Vent_amplitude;
      PACE_GND_CTRL = true;
      ATR_PACE_CTRL = false;
      Z_ATR_CTRL = false;
      Z_VENT_CTRL = false;
      VENT_PACE_CTRL = false;
      VENT_GND_CTRL = false;
      ATR_GND_CTRL = true;
      PACE_CHARGE_CTRL = true;
    state DOO_PACE_VENT
      entry:
      LED_green = true;
      PACE_CHARGE_CTRL = false;
      PACE_GND_CTRL = true;
      ATR_PACE_CTRL = false;
      ATR_GND_CTRL = false;
      Z_ATR_CTRL = false;
      Z_VENT_CTRL = false;
      VENT_GND_CTRL = false;
      VENT_PACE_CTRL = true;
    VOO_DischargeC21A_ChargeC22V -> DOO_PACE_ATRIUM [order 1] : after(Lower_period-(AV_delay+Vent_pulse_width), msec)
    DOO_PACE_ATRIUM -> DOO_DischargeC21A_ChargeC22V : after(Atrial_pulse_width, msec)
    DOO_PACE_VENT -> VOO_DischargeC21A_ChargeC22V : after(Vent_pulse_width, msec)
    DOO_DischargeC21A_ChargeC22V -> DOO_PACE_VENT : after(AV_delay - Atrial_pulse_width, msec)
  AOO_DischargeC21_ChargeC22 -> HOLD [order 2] : [MODE~=1]
  VOO_DischargeC21_ChargeC22 -> HOLD [order 2] : [MODE~=2]
  AAI.AAI_DischargeC21_ChargeC22 -> HOLD [order 3] : [MODE~=3]
  VVI.VVI_DischargeC21_ChargeC22 -> HOLD [order 3] : [MODE~=4]
  VOO_DischargeC21A_ChargeC22V -> HOLD [order 2] : [MODE~=5]
  HOLD -> VOO_DischargeC21A_ChargeC22V [order 6] : [MODE==5]
  HOLD -> AAI.AAI_DischargeC21_ChargeC22 [order 3] : [MODE==3]
  HOLD -> VVI.VVI_DischargeC21_ChargeC22 [order 5] : [MODE==4]
  HOLD -> VOO_DischargeC21_ChargeC22 [order 4] : [MODE==2]
  HOLD -> AOO_DischargeC21_ChargeC22 [order 2] : [MODE==1]
  (default) -> HOLD
  HOLD -> HOLD [order 1] : [MODE==0 || Lower_rate_limit>Upper_rate_limit]
  data: PACE_amplitude output double; MODE input uint8; Atrial_amplitude input double; Vent_amplitude input double; Lower_period input uint16; Lower_rate_limit input uint16; Upper_rate_limit input uint16; Atrial_pulse_width input uint16; PACE_CHARGE_CTRL output boolean; ATR_PACE_CTRL output boolean; ATR_GND_CTRL output boolean; Z_ATR_CTRL output boolean; VENT_PACE_CTRL output boolean; VENT_GND_CTRL output boolean; Z_VENT_CTRL output boolean; PACE_GND_CTRL output boolean; FRONTEND_CTRL output boolean; LED_red output boolean; LED_green output boolean; LED_blue output boolean; Vent_pulse_width input uint16; ARP input uint16; VRP input uint16; AV_delay input uint16; ATR_CMP_DETECT input boolean; VENT_CMP_DETECT input boolean; APW_delay local uint16; VPW_delay local uint16; Period_R input uint16
